simulink model "amortiguador (1)"  (R2022b)
settings: Solver=VariableStepAuto  StartTime=0.0  StopTime=10  MaxStep=1  RelTol=1e-3
values from neighbouring files (symbols this model uses):
  b1 = 1000    [DobleP1.m]
  k1 = 16182    [DobleP1.m]
  k2 = 19000    [DobleP1.m]
  m1 = 290    [DobleP1.m]
settings Model: Creator=bryan  LastModifiedBy=bryan

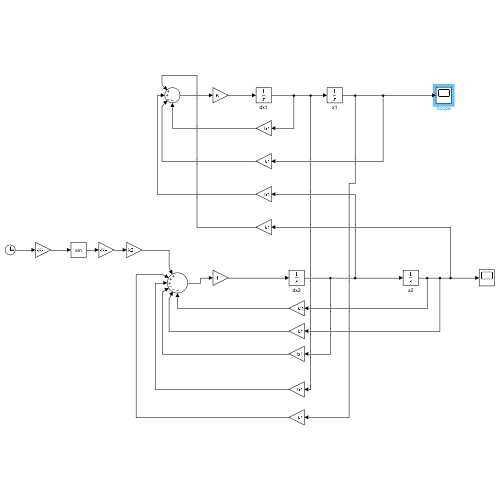
[thumbnail: Simulink's stored preview of the top-level diagram]
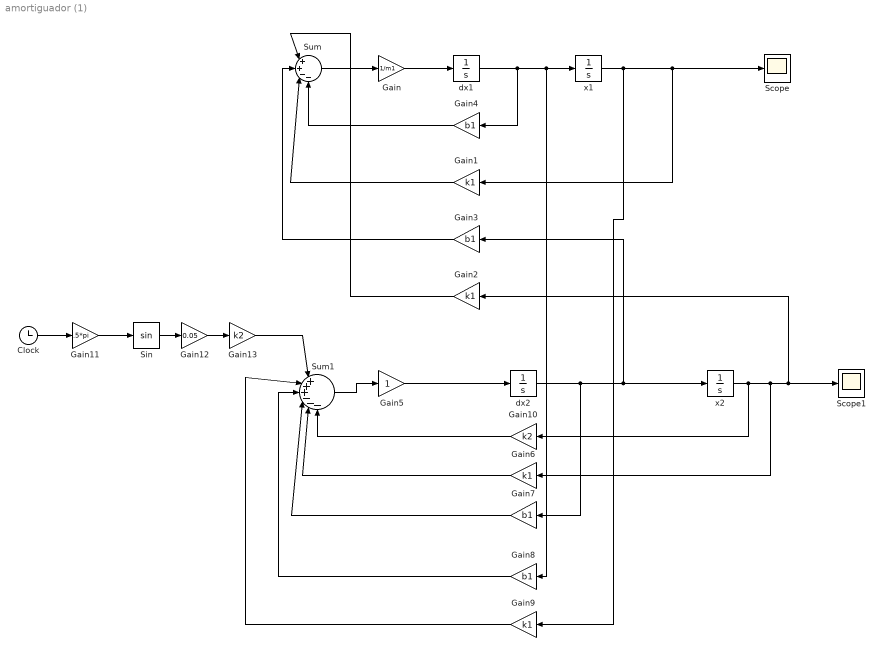
== system amortiguador (1) ==
  Clock : Clock
  Gain : Gain  Gain=1/m1
  Gain{1..2,6,9} (4 alike) : Gain  Gain=k1
  Gain10 : Gain  Gain=k2
  Gain11 : Gain  Gain=.5*pi
  Gain12 : Gain  Gain=0.05
  Gain13 : Gain  Gain=k2
  Gain{3..4,7..8} (4 alike) : Gain  Gain=b1
  Gain5 : Gain
  Scope : Scope
  Scope1 : Scope
  Sin : Trigonometry
  Sum : Sum  Inputs=|++--
  Sum1 : Sum  Inputs=|+++---
  dx1 : Integrator
  dx2 : Integrator
  x1 : Integrator
  x2 : Integrator
  wires:
  dx1/1 -> Gain4/1, Gain8/1, x1/1
  x1/1 -> Gain9/1, Scope/1, Gain1/1
  Sum/1 -> Gain/1
  Gain/1 -> dx1/1
  Gain4/1 -> Sum/4
  Gain1/1 -> Sum/3
  Gain3/1 -> Sum/2
  Gain2/1 -> Sum/1
  dx2/1 -> Gain7/1, Gain3/1, x2/1
  Gain5/1 -> dx2/1
  Sum1/1 -> Gain5/1
  Gain10/1 -> Sum1/6
  Gain6/1 -> Sum1/5
  Gain8/1 -> Sum1/3
  Gain7/1 -> Sum1/4
  Gain9/1 -> Sum1/2
  x2/1 -> Gain10/1, Gain6/1, Scope1/1, Gain2/1
  Clock/1 -> Gain11/1
  Gain11/1 -> Sin/1
  Sin/1 -> Gain12/1
  Gain12/1 -> Gain13/1
  Gain13/1 -> Sum1/1
